simulink model "mode10"  (R2021a)
settings: Solver=VariableStepAuto  StartTime=0.0  StopTime=20  RelTol=1e-3
libraries: simulink_extras x4
settings Model: Creator=DELL  LastModifiedBy=DELL

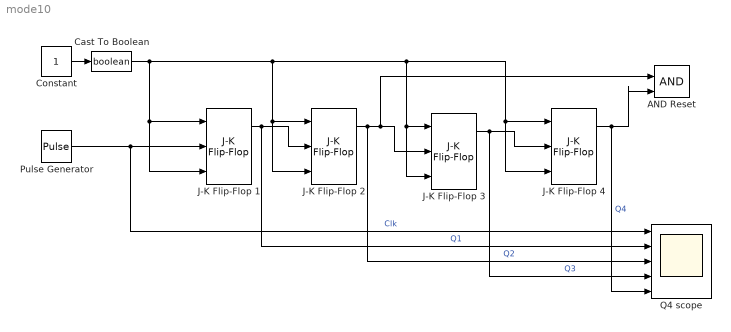
== system mode10 ==
  AND Reset : Logic  IconShape=distinctive  AllPortsSameDT=off  OutDataTypeStr=boolean
  Cast To Boolean : DataTypeConversion  OutDataTypeStr=boolean
  Constant : Constant
  J-K Flip-Flop {1..4} (4 alike) : simulink_extras/Flip Flops/J-K Flip-Flop  initial_condition=0
  Pulse Generator : DiscretePulseGenerator  PulseType=Time based  Period=1  PulseWidth=5
  Q4 scope : Scope  NumInputPorts=5
  wires:
  Pulse Generator/1 -> Q4 scope/1, J-K Flip-Flop 1/2  "Clk"
  J-K Flip-Flop 1/1 -> Q4 scope/2, J-K Flip-Flop 2/2  "Q1"
  J-K Flip-Flop 2/1 -> Q4 scope/3, AND Reset/1, J-K Flip-Flop 3/2  "Q2"
  J-K Flip-Flop 3/1 -> Q4 scope/4, J-K Flip-Flop 4/2  "Q3"
  J-K Flip-Flop 4/1 -> Q4 scope/5, AND Reset/2  "Q4"
  Cast To Boolean/1 -> J-K Flip-Flop 2/1, J-K Flip-Flop 2/3, J-K Flip-Flop 3/1, J-K Flip-Flop 3/3, J-K Flip-Flop 4/1, J-K Flip-Flop 4/3, J-K Flip-Flop 1/1, J-K Flip-Flop 1/3
  Constant/1 -> Cast To Boolean/1
